simulink model "NUgus"  (R2018a)
settings: Solver=VariableStepAuto  StartTime=0.0  StopTime=inf  RelTol=1e-2
values from neighbouring files (symbols this model uses):
  CM740_acc_bias = 4 * 9.80743    (= 39.22972)    [CM740_init.m]
  CM740_acc_gain = 512 / CM740_acc_centre    [CM740_init.m]
  CM740_gyro_bias = 1600 / 360 * 2 * pi    (= 27.9252680319)    [CM740_init.m]
  CM740_gyro_gain = 512 / CM740_gyro_centre    [CM740_init.m]
  g = 9.8107    [init.m]
  head = [-0.05482228998067195, -0.00010888238321339966, 0.0011712900228573724, 0.41900000000000004]    [comtest.m]
  Kw = 0.9    [init.m]
  model = NUgusKinematics()    [KinematicsTest.m]    (also in Support_Region.m; init.m = NUgusKinematics)
  period = 1.0    (= 1)    [init.m]
  s = mean(abs(present_speed.data))    [RunServoTest.m]
  sample_time = 1/90    (= 0.0111111111111)    [init.m]
  step_height = 0.1    [init.m]
  torso = [0.0050079703254699804, 0.008880921777563762, 0.1021503146237477, 2.5390000000000006]    [comtest.m]
  z0 = 0.45    [init.m]
undefined symbols (not defined in the file or in its folder): sigbuilder_block, X, Y, Z
libraries: sm_lib x206, nesl_utility x82, Contact_Forces_Lib x10
(part 7 of 7)

== system NUgus/NUgus/6 DoF/to IMU ==
  alpha : Inport
  omega : Inport  Port=2
  Rtw : Inport  Port=3
  Data Store Write : DataStoreWrite  DataStoreName=CM740  SampleTime=sample_time  DataStoreElements=CM740.acc_x#CM740.acc_y#CM740.acc_z#CM740.gyro_x#CM740.gyro_y#CM740.gyro_z
  IMU : Subsystem
  wires:
  IMU/3(alphaz) -> Data Store Write/3
  IMU/2(alphay) -> Data Store Write/2
  IMU/1(alphax) -> Data Store Write/1
  IMU/4(omegax) -> Data Store Write/4
  IMU/6(omegaz) -> Data Store Write/6
  Rtw/1 -> IMU/1(Rtw)
  omega/1 -> IMU/2(w)
  alpha/1 -> IMU/3(a)
  IMU/5(omegay) -> Data Store Write/5

== system NUgus/NUgus/IMU1/Convert Acc ==
  PS-Simulink Converter{,1..3} (4 alike) : nesl_utility/PS-Simulink Converter  PhysicalDomain=network_engine_domain  SubClassName=ps_output  LeftPortType=input  RightPortType=output  PseudoPeriodic=off  Frequencies=[]  Unit=1  AffineConversion=off
  Ha : PMIOPort  Side=Left
  x : PMIOPort  Port=2  Side=Left
  y : PMIOPort  Port=3  Side=Left
  z : PMIOPort  Port=4  Side=Left
  Htw : Outport
  ax : Outport  Port=2
  ay : Outport  Port=3
  az : Outport  Port=4
  wires:
  PS-Simulink Converter2/1 -> az/1
  PS-Simulink Converter1/1 -> ay/1
  PS-Simulink Converter/1 -> ax/1
  PS-Simulink Converter3/1 -> Htw/1
  connections:
  PS-Simulink Converter2/LConn1 -- z/RConn1
  PS-Simulink Converter/LConn1 -- x/RConn1
  PS-Simulink Converter1/LConn1 -- y/RConn1
  Ha/RConn1 -- PS-Simulink Converter3/LConn1

== system NUgus/NUgus/IMU1/Convert Gyro ==
  PS-Simulink Converter : nesl_utility/PS-Simulink Converter  PhysicalDomain=network_engine_domain  SubClassName=ps_output  LeftPortType=input  RightPortType=output  PseudoPeriodic=off  Frequencies=[]  Unit=rad/s  AffineConversion=off
  PS-Simulink Converter1 : nesl_utility/PS-Simulink Converter  PhysicalDomain=network_engine_domain  SubClassName=ps_output  LeftPortType=input  RightPortType=output  PseudoPeriodic=off  Frequencies=[]  Unit=rad/s  AffineConversion=off
  PS-Simulink Converter2 : nesl_utility/PS-Simulink Converter  PhysicalDomain=network_engine_domain  SubClassName=ps_output  LeftPortType=input  RightPortType=output  PseudoPeriodic=off  Frequencies=[]  Unit=rad/s  AffineConversion=off
  x : PMIOPort  Side=Left
  y : PMIOPort  Port=2  Side=Left
  z : PMIOPort  Port=3  Side=Left
  wx : Outport
  wy : Outport  Port=2
  wz : Outport  Port=3
  wires:
  PS-Simulink Converter2/1 -> wz/1
  PS-Simulink Converter1/1 -> wy/1
  PS-Simulink Converter/1 -> wx/1
  connections:
  PS-Simulink Converter2/LConn1 -- z/RConn1
  PS-Simulink Converter/LConn1 -- x/RConn1
  PS-Simulink Converter1/LConn1 -- y/RConn1

== system NUgus/NUgus/IMU1/Saturate Acc ==
  Hta : Inport
  Acc : Inport  Port=2
  Acc Saturation : Saturate  UpperLimit=1023  LowerLimit=0
  Add : Sum  Inputs=+++
  Constant : Constant  Value=CM740_acc_bias
  Constant1 : Constant  Value=[0 0 9.80743]
  Gain : Gain  Gain=[0 0 1]
  Gain1 : Gain  Gain=CM740_acc_gain  OutDataTypeStr=int16
  Matrix Multiply : Product  Multiplication=Matrix(*)
  Transpose : Math  Operator=transpose  SaturateOnIntegerOverflow=on
  alpha : Outport
  wires:
  Acc/1 -> Add/3
  Add/1 -> Gain1/1
  Acc Saturation/1 -> alpha/1
  Gain/1 -> Add/1
  Gain1/1 -> Acc Saturation/1
  Constant/1 -> Add/2
  Transpose/1 -> Matrix Multiply/1
  Hta/1 -> Transpose/1
  Constant1/1 -> Matrix Multiply/2
  Matrix Multiply/1 -> Gain/1

== system NUgus/NUgus/IMU1/Saturate Gyro ==
  w : Inport
  Add1 : Sum
  Constant1 : Constant  Value=CM740_gyro_bias
  Gain : Gain  Gain=CM740_gyro_gain  OutDataTypeStr=int16
  Gyro Saturation : Saturate  UpperLimit=1023  LowerLimit=0
  omega : Outport
  wires:
  Constant1/1 -> Add1/2
  Gyro Saturation/1 -> omega/1
  Add1/1 -> Gain/1
  Gain/1 -> Gyro Saturation/1
  w/1 -> Add1/1

== system NUgus/NUgus/left_foot/foot ==
  Inertia : sm_lib/Body Elements/Inertia  InertiaType=Custom  Mass=model.mass.foot(4)  MassUnits=kg  CenterOfMass=[0, 0, 0]  CenterOfMassUnits=m  MomentsOfInertia=[model.inertia.foot(1,1), model.inertia.foot(2,2), model.inertia.foot(3,3)]  MomentsOfInertiaUnits=kg*m^2  ProductsOfInertia=-[model.inertia.foot(2,3), -model.inertia.foot(3,1), -model.inertia.foot(1,2)]  ProductsOfInertiaUnits=kg*m^2  GraphicType=Marker  MarkerShape=Inertia  MarkerSize=20  GraphicVisPropType=SimpleVisualProperties  GraphicDiffuseColor=[0.8 0.8 0.8]  GraphicSpecularColor=[0.5 0.5 0.5 1.0]  GraphicAmbientColor=[0.15 0.15 0.15 1.0]  GraphicEmissiveColor=[0.0 0.0 0.0 1.0]  GraphicShininess=75  GraphicOpacity=inertia_opacity
  InertiaOriginTransform : sm_lib/Frames and Transforms/Rigid Transform  TranslationMethod=Cartesian  TranslationStandardOffset=0  TranslationLengthUnit=m  TranslationStandardAxis=+Z  TranslationCartesianOffset=[-0.007551 -0.077046 -0.031619]  TranslationROffset=0  TranslationROffsetUnits=m  TranslationZOffset=0  TranslationZOffsetUnits=m  TranslationThetaOffset=0  TranslationThetaOffsetUnits=deg  RotationMethod=RotationSequence  RotationAngleUnits=deg  RotationStandardAxis=+Z  RotationAngle=0.0  RotationArbitraryAxis=[0 0 1]  FollAlignAxisA=+X  BaseAlignAxisA=+Y  FollAlignAxisB=+Y  BaseAlignAxisB=+Z  RotationSequenceAxes=BaseAxes  RotationSequence=XYZ  RotationSequenceAngles=[0, 0, 0]  RotationSequenceAnglesUnits=rad  RotationMatrix=[1 0 0; 0 1 0; 0 0 1]
  ReferenceFrame : sm_lib/Frames and Transforms/Reference Frame
  right_ankle_roll_AxisInvTransform : sm_lib/Frames and Transforms/Rigid Transform  TranslationMethod=Cartesian  TranslationStandardOffset=0  TranslationLengthUnit=m  TranslationStandardAxis=+Z  TranslationCartesianOffset=[0, 0, 0]  TranslationROffset=0  TranslationROffsetUnits=m  TranslationZOffset=0  TranslationZOffsetUnits=m  TranslationThetaOffset=0  TranslationThetaOffsetUnits=deg  RotationMethod=ArbitraryAxis  RotationAngleUnits=rad  RotationStandardAxis=+Z  RotationAngle=1.570796326794897  RotationArbitraryAxis=[1, 0, 0]  FollAlignAxisA=+X  BaseAlignAxisA=+Y  FollAlignAxisB=+Y  BaseAlignAxisB=+Z  RotationSequenceAxes=FollowerAxes  RotationSequence=XYX  RotationSequenceAngles=[0 0 0]  RotationSequenceAnglesUnits=deg  RotationMatrix=[1 0 0; 0 1 0; 0 0 1]
  right_foot_visual : sm_lib/Body Elements/Solid  InertiaType=Custom  Mass=0  MassUnits=kg  CenterOfMass=[0, 0, 0]  CenterOfMassUnits=m  MomentsOfInertia=[0, 0, 0]  MomentsOfInertiaUnits=kg*m^2  ProductsOfInertia=[0, 0, 0]  ProductsOfInertiaUnits=kg*m^2  DensityBased=on  Density=1000  DensityUnits=kg/m^3  DoExposeReferenceFrame=on  SerializedFrames=<Frames/>  GraphicType=FromGeometry  MarkerShape=Sphere  MarkerSize=10  GraphicVisPropType=SimpleVisualProperties  GraphicDiffuseColor=[0.5, 0.5, 0.5]  GraphicSpecularColor=[0.5 0.5 0.5 1.0]  GraphicAmbientColor=[0.15 0.15 0.15 1.0]  GraphicEmissiveColor=[0.0 0.0 0.0 1.0]  GraphicShininess=75  GraphicOpacity=1  GeometryShape=FromFile  RectangleSize=[1 1]  RectangleSizeUnits=m  BrickDimensions=[1 1 1]  BrickDimensionUnits=m  CylinderRadius=1  CylinderRadiusUnits=m  CylinderLength=1  CylinderLengthUnits=m  SphereRadius=1  SphereRadiusUnits=m  EllipsoidRadii=[1 1 1]  EllipsoidRadiiUnits=m  ExtrusionCrossSection=[1 1; -1 1; -1 -1; 1 -1]  ExtrusionCrossSectionUnits=m  ExtrusionLength=1  ExtrusionLengthUnits=m  PolygonNumSides=3  PolygonOuterRadius=1  PolygonOuterRadiusUnits=m  ExtGeomFileType=STL  ExtGeomFileName=mesh/left_foot.stl  ExtGeomFileUnits=m  RevolutionCrossSection=[1 1; 1 -1; 2 -1; 2 1]  RevolutionCrossSectionUnits=m  RevolutionExtent=Full  RevolutionAngle=180  RevolutionAngleUnits=deg
  right_foot_visualOriginTransform : sm_lib/Frames and Transforms/Rigid Transform  TranslationMethod=Cartesian  TranslationStandardOffset=0  TranslationLengthUnit=m  TranslationStandardAxis=+Z  TranslationCartesianOffset=[0, 0, 0]  TranslationROffset=0  TranslationROffsetUnits=m  TranslationZOffset=0  TranslationZOffsetUnits=m  TranslationThetaOffset=0  TranslationThetaOffsetUnits=deg  RotationMethod=RotationSequence  RotationAngleUnits=deg  RotationStandardAxis=+Z  RotationAngle=0.0  RotationArbitraryAxis=[0 0 1]  FollAlignAxisA=+X  BaseAlignAxisA=+Y  FollAlignAxisB=+Y  BaseAlignAxisB=+Z  RotationSequenceAxes=BaseAxes  RotationSequence=XYZ  RotationSequenceAngles=[0, 0, 0]  RotationSequenceAnglesUnits=rad  RotationMatrix=[1 0 0; 0 1 0; 0 0 1]
  F : PMIOPort  Side=Left
  B : PMIOPort  Port=2  Side=Right
  connections:
  Inertia/RConn1 -- InertiaOriginTransform/RConn1
  ReferenceFrame/RConn1 -- InertiaOriginTransform/LConn1 -- right_ankle_roll_AxisInvTransform/LConn1 -- right_foot_visualOriginTransform/LConn1 -- B/RConn1
  right_ankle_roll_AxisInvTransform/RConn1 -- F/RConn1
  right_foot_visual/RConn1 -- right_foot_visualOriginTransform/RConn1

== system NUgus/NUgus/right_foot/foot ==
  Inertia : sm_lib/Body Elements/Inertia  InertiaType=Custom  Mass=model.mass.foot(4)  MassUnits=kg  CenterOfMass=[0, 0, 0]  CenterOfMassUnits=m  MomentsOfInertia=[model.inertia.foot(1,1), model.inertia.foot(2,2), model.inertia.foot(3,3)]  MomentsOfInertiaUnits=kg*m^2  ProductsOfInertia=-[model.inertia.foot(2,3), model.inertia.foot(3,1), model.inertia.foot(1,2)]  ProductsOfInertiaUnits=kg*m^2  GraphicType=Marker  MarkerShape=Inertia  MarkerSize=20  GraphicVisPropType=SimpleVisualProperties  GraphicDiffuseColor=[0.8 0.8 0.8]  GraphicSpecularColor=[0.5 0.5 0.5 1.0]  GraphicAmbientColor=[0.15 0.15 0.15 1.0]  GraphicEmissiveColor=[0.0 0.0 0.0 1.0]  GraphicShininess=75  GraphicOpacity=inertia_opacity
  InertiaOriginTransform : sm_lib/Frames and Transforms/Rigid Transform  TranslationMethod=Cartesian  TranslationStandardOffset=0  TranslationLengthUnit=m  TranslationStandardAxis=+Z  TranslationCartesianOffset=[-0.007551 -0.077046 -0.031619]  TranslationROffset=0  TranslationROffsetUnits=m  TranslationZOffset=0  TranslationZOffsetUnits=m  TranslationThetaOffset=0  TranslationThetaOffsetUnits=deg  RotationMethod=RotationSequence  RotationAngleUnits=deg  RotationStandardAxis=+Z  RotationAngle=0.0  RotationArbitraryAxis=[0 0 1]  FollAlignAxisA=+X  BaseAlignAxisA=+Y  FollAlignAxisB=+Y  BaseAlignAxisB=+Z  RotationSequenceAxes=BaseAxes  RotationSequence=XYZ  RotationSequenceAngles=[0, 0, 0]  RotationSequenceAnglesUnits=rad  RotationMatrix=[1 0 0; 0 1 0; 0 0 1]
  ReferenceFrame : sm_lib/Frames and Transforms/Reference Frame
  right_ankle_roll_AxisInvTransform : sm_lib/Frames and Transforms/Rigid Transform  TranslationMethod=Cartesian  TranslationStandardOffset=0  TranslationLengthUnit=m  TranslationStandardAxis=+Z  TranslationCartesianOffset=[0, 0, 0]  TranslationROffset=0  TranslationROffsetUnits=m  TranslationZOffset=0  TranslationZOffsetUnits=m  TranslationThetaOffset=0  TranslationThetaOffsetUnits=deg  RotationMethod=ArbitraryAxis  RotationAngleUnits=rad  RotationStandardAxis=+Z  RotationAngle=1.570796326794897  RotationArbitraryAxis=[1, 0, 0]  FollAlignAxisA=+X  BaseAlignAxisA=+Y  FollAlignAxisB=+Y  BaseAlignAxisB=+Z  RotationSequenceAxes=FollowerAxes  RotationSequence=XYX  RotationSequenceAngles=[0 0 0]  RotationSequenceAnglesUnits=deg  RotationMatrix=[1 0 0; 0 1 0; 0 0 1]
  right_foot_visual : sm_lib/Body Elements/Solid  InertiaType=Custom  Mass=0  MassUnits=kg  CenterOfMass=[0, 0, 0]  CenterOfMassUnits=m  MomentsOfInertia=[0, 0, 0]  MomentsOfInertiaUnits=kg*m^2  ProductsOfInertia=[0, 0, 0]  ProductsOfInertiaUnits=kg*m^2  DensityBased=on  Density=1000  DensityUnits=kg/m^3  DoExposeReferenceFrame=on  SerializedFrames=<Frames/>  GraphicType=FromGeometry  MarkerShape=Sphere  MarkerSize=10  GraphicVisPropType=SimpleVisualProperties  GraphicDiffuseColor=[0.5, 0.5, 0.5]  GraphicSpecularColor=[0.5 0.5 0.5 1.0]  GraphicAmbientColor=[0.15 0.15 0.15 1.0]  GraphicEmissiveColor=[0.0 0.0 0.0 1.0]  GraphicShininess=75  GraphicOpacity=1  GeometryShape=FromFile  RectangleSize=[1 1]  RectangleSizeUnits=m  BrickDimensions=[1 1 1]  BrickDimensionUnits=m  CylinderRadius=1  CylinderRadiusUnits=m  CylinderLength=1  CylinderLengthUnits=m  SphereRadius=1  SphereRadiusUnits=m  EllipsoidRadii=[1 1 1]  EllipsoidRadiiUnits=m  ExtrusionCrossSection=[1 1; -1 1; -1 -1; 1 -1]  ExtrusionCrossSectionUnits=m  ExtrusionLength=1  ExtrusionLengthUnits=m  PolygonNumSides=3  PolygonOuterRadius=1  PolygonOuterRadiusUnits=m  ExtGeomFileType=STL  ExtGeomFileName=mesh/right_foot.stl  ExtGeomFileUnits=m  RevolutionCrossSection=[1 1; 1 -1; 2 -1; 2 1]  RevolutionCrossSectionUnits=m  RevolutionExtent=Full  RevolutionAngle=180  RevolutionAngleUnits=deg
  right_foot_visualOriginTransform : sm_lib/Frames and Transforms/Rigid Transform  TranslationMethod=Cartesian  TranslationStandardOffset=0  TranslationLengthUnit=m  TranslationStandardAxis=+Z  TranslationCartesianOffset=[0, 0, 0]  TranslationROffset=0  TranslationROffsetUnits=m  TranslationZOffset=0  TranslationZOffsetUnits=m  TranslationThetaOffset=0  TranslationThetaOffsetUnits=deg  RotationMethod=RotationSequence  RotationAngleUnits=deg  RotationStandardAxis=+Z  RotationAngle=0.0  RotationArbitraryAxis=[0 0 1]  FollAlignAxisA=+X  BaseAlignAxisA=+Y  FollAlignAxisB=+Y  BaseAlignAxisB=+Z  RotationSequenceAxes=BaseAxes  RotationSequence=XYZ  RotationSequenceAngles=[0, 0, 0]  RotationSequenceAnglesUnits=rad  RotationMatrix=[1 0 0; 0 1 0; 0 0 1]
  F : PMIOPort  Side=Left
  B : PMIOPort  Port=2  Side=Right
  connections:
  Inertia/RConn1 -- InertiaOriginTransform/RConn1
  ReferenceFrame/RConn1 -- InertiaOriginTransform/LConn1 -- B/RConn1 -- right_ankle_roll_AxisInvTransform/LConn1 -- right_foot_visualOriginTransform/LConn1
  right_ankle_roll_AxisInvTransform/RConn1 -- F/RConn1
  right_foot_visual/RConn1 -- right_foot_visualOriginTransform/RConn1

== system NUgus/NUgus/6 DoF/to IMU/IMU ==
  Rtw : Inport
  w : Inport  Port=2
  a : Inport  Port=3
  Demux : Demux  Outputs=3
  Demux1 : Demux  Outputs=3
  IMU Continuous : Scope  NumInputPorts=2
  IMU Discrete : Scope  NumInputPorts=2
  Saturate Acc : Subsystem
  Saturate Gyro : Subsystem
  alphax : Outport
  alphay : Outport  Port=2
  alphaz : Outport  Port=3
  omegax : Outport  Port=4
  omegay : Outport  Port=5
  omegaz : Outport  Port=6
  wires:
  Demux/1 -> omegax/1
  Demux/2 -> omegay/1
  Demux/3 -> omegaz/1
  Demux1/3 -> alphaz/1
  Demux1/1 -> alphax/1
  Demux1/2 -> alphay/1
  Saturate Acc/1(alpha) -> IMU Discrete/2, Demux1/1
  w/1 -> IMU Continuous/1, Saturate Gyro/1(w)
  Saturate Gyro/1(omega) -> IMU Discrete/1, Demux/1
  a/1 -> Saturate Acc/2(Acc), IMU Continuous/2
  Rtw/1 -> Saturate Acc/1(Rtw)

== system NUgus/NUgus/6 DoF/to IMU/IMU/Saturate Acc ==
  Rtw : Inport
  Acc : Inport  Port=2
  Acc Saturation : Saturate  UpperLimit=1023  LowerLimit=0
  Add : Sum  Inputs=+++
  Constant : Constant  Value=CM740_acc_bias
  Constant1 : Constant  Value=[0 0 9.80743]
  Gain : Gain  Gain=[1 1 -1]
  Gain1 : Gain  Gain=CM740_acc_gain  OutDataTypeStr=int16
  Matrix Multiply : Product  Multiplication=Matrix(*)
  Transpose : Math  Operator=transpose  SaturateOnIntegerOverflow=on
  alpha : Outport
  wires:
  Acc/1 -> Add/3
  Add/1 -> Gain1/1
  Acc Saturation/1 -> alpha/1
  Gain/1 -> Add/1
  Gain1/1 -> Acc Saturation/1
  Constant/1 -> Add/2
  Transpose/1 -> Matrix Multiply/1
  Rtw/1 -> Transpose/1
  Constant1/1 -> Matrix Multiply/2
  Matrix Multiply/1 -> Gain/1

== system NUgus/NUgus/6 DoF/to IMU/IMU/Saturate Gyro ==
  w : Inport
  Add1 : Sum
  Constant1 : Constant  Value=CM740_gyro_bias
  Gain : Gain  Gain=CM740_gyro_gain  OutDataTypeStr=int16
  Gyro Saturation : Saturate  UpperLimit=1023  LowerLimit=0
  omega : Outport
  wires:
  Constant1/1 -> Add1/2
  Gyro Saturation/1 -> omega/1
  Add1/1 -> Gain/1
  Gain/1 -> Gyro Saturation/1
  w/1 -> Add1/1

== matlab function NUgus/Kinematics/Forward Kinematics/Simulink Function/FK Function ==
  data: HtRSp output; p input; HtLSp output; HtRSr output; HtLSr output; HtRE output; HtLE output; HtRHy output; HtLHy output; HtRHr output; HtLHr output; HtRHp output; HtLHp output; HtRK output; HtLK output; HtRAp output; HtLAp output; HtRAr output; HtLAr output; HtHy output; HtHp output
function [HtRSp, HtLSp, HtRSr, HtLSr, HtRE, HtLE, HtRHy, HtLHy, HtRHr, HtLHr, HtRHp, HtLHp, HtRK, HtLK, HtRAp, HtLAp, HtRAr, HtLAr, HtHy, HtHp] = FK(p)
    model = NUgusKinematics();

    kinematics = Kinematics(model);
    
    % Get FK for arms
    [RSp, RSr, RE] = kinematics.armFK(p, false);
    [LSp, LSr, LE] = kinematics.armFK(p, true);
    % Get FK for legs
    [RHy, RHr, RHp, RK, RAp, RAr] = kinematics.legFK(p, false);
    [LHy, LHr, LHp, LK, LAp, LAr] = kinematics.legFK(p, true);
    % Get FK for Head
    [Hy, Hp] = kinematics.headFK(p);
    
    % Return FK in servo order
    HtRSp = RSp.tf;
    HtLSp = LSp.tf;
    
    HtRSr = RSr.tf;
    HtLSr = LSr.tf;
    
    HtRE = RE.tf;
    HtLE = LE.tf;
    
    HtRHy = RHy.tf;
    HtLHy = LHy.tf;
    
    HtRHr = RHr.tf;
    HtLHr = LHr.tf;
    
    HtRHp = RHp.tf;
    HtLHp = LHp.tf;
    
    HtRK = RK.tf;
    HtLK = LK.tf;
    
    HtRAp = RAp.tf;
    HtLAp = LAp.tf;
    
    HtRAr = RAr.tf;
    HtLAr = LAr.tf;
    
    HtHy = Hy.tf;
    HtHp = Hp.tf;
end

== matlab function NUgus/Kinematics/Centre of Mass/Simulink Function/COM Function ==
  data: HtRSp input; HtLSp input; HtRSr input; HtLSr input; HtRE input; HtLE input; HtRHy input; HtLHy input; HtRHr input; HtLHr input; HtRHp input; HtLHp input; HtRK input; HtLK input; HtRAp input; HtLAp input; HtRAr input; HtLAr input; HtHy input; HtHp input; com output; mass output
function [com, mass] = COM(HtRSp, HtLSp, HtRSr, HtLSr, HtRE, HtLE, HtRHy, HtLHy, HtRHr, HtLHr, HtRHp, HtLHp, HtRK, HtLK, HtRAp, HtLAp, HtRAr, HtLAr, HtHy, HtHp)
    model = NUgusKinematics();
    
    % Store mass particles and their transforms to multiply
    ms = [model.mass.head; model.mass.arm_upper; model.mass.arm_upper; model.mass.arm_lower; model.mass.arm_lower; model.mass.hip_block; model.mass.hip_block; model.mass.leg_upper; model.mass.leg_upper; model.mass.leg_lower; model.mass.leg_lower; model.mass.ankle_block; model.mass.ankle_block; model.mass.foot; model.mass.foot; model.mass.torso];
    tf = [HtHp, HtRSp, HtLSp, HtRSr, HtLSr, HtRHr, HtLHr, HtRHp, HtLHp, HtRK, HtLK, HtRAp, HtLAp, HtRAr, HtLAr, [1 0 0 0; 0 1 0 0; 0 0 1 0; 0 0 0 1]];

    % Store CoM as x,y,z coordinates
    com = [0; 0; 0];
    mass = 0;

    for ii=1:size(ms, 1)
        % Get transform of the particle
        t = tf(1:4, ii*4-3:ii*4);
        % Alias particle CoM and mass for convenience
        p_com  = [ms(ii, 1:3) 1]';
        p_com  = t * p_com;
        p_mass = ms(ii, 4);
        % Calculate new CoM and updated mass
        com = (com * mass + p_com(1:3) * p_mass) / (mass + p_mass);
        mass = mass + p_mass;
    end
    
end

== matlab function NUgus/Simulink Function/MATLAB Function ==
  data: x input; H output; y input; z input; roll input; pitch input; yaw input
function H = getTransform(x,y,z,roll,pitch,yaw)
    t = Transform3D();    
    t = t.translate([x,y,z]).rotateX(roll).rotateY(pitch).rotateZ(yaw);
    H = t.tf;
end

== matlab function NUgus/Kinematics/Inverse Kinematics/Simulink Function/IK Function ==
  data: thetaTRSp output; rTRh input; rTLh input; HTRl input; HTLl input; rCP input; thetaTLSp output; thetaTRSr output; thetaTLSr output; thetaTRE output; thetaTLE output; thetaTRHy output; thetaTLHy output; thetaTRHr output; thetaTLHr output; thetaTRHp output; thetaTLHp output; thetaTRK output; thetaTLK output; thetaTRAp output; thetaTLAp output; thetaTRAr output; thetaTLAr output; thetaTNy output; thetaTNp output
function [thetaTRSp, thetaTLSp, thetaTRSr, thetaTLSr, thetaTRE, thetaTLE, thetaTRHy, thetaTLHy, thetaTRHr, thetaTLHr, thetaTRHp, thetaTLHp, thetaTRK, thetaTLK, thetaTRAp, thetaTLAp, thetaTRAr, thetaTLAr, thetaTNy, thetaTNp] = IK(rTRh, rTLh, HTRl, HTLl, rCP)
    model = NUgusKinematics();

    kinematics = Kinematics(model);

    % Head IK
    [thetaTNy, thetaTNp] = kinematics.headIK(rCP);
    
    % Arm IK
    [thetaTRSp, thetaTRSr, thetaTRE] = kinematics.armIK(rTRh, false);
    [thetaTLSp, thetaTLSr, thetaTLE] = kinematics.armIK(rTLh, true);
    
    % Leg IK
    [thetaTRHy, thetaTRHr, thetaTRHp, thetaTRK, thetaTRAp, thetaTRAr] = kinematics.legIK(HTRl, false);
    [thetaTLHy, thetaTLHr, thetaTLHp, thetaTLK, thetaTLAp, thetaTLAr] = kinematics.legIK(HTLl, true);
end

== stateflow chart NUgus/Control/Step Logic ==
  settings: updateMethod=DISCRETE  sampleTime=0.1  initializeOutput=1
  state update [function]
    (default) -> (junction 109) : {
        | %Update right
        | xr = xr + Kw*(xr_ref - xr);
        | yr = yr + Kw*(yr_ref - yr);
        | zr = zr + Kw*(zr_ref - zr);
        | % Update left
        | xl = xl + Kw*(xl_ref - xl);
        | yl = yl + Kw*(yl_ref - yl);
        | zl = zl + Kw*(zl_ref - zl);
        | % Store updates
        | rfoot = [xr; yr; zr];
        | lfoot = [xl; yl; zl];
        | }
  state RightSwing
    % Right foot swing
    % Left foot support
    en, du:
    update;
    state Right [parallel]
      en,du:
      % Left support
      zl_ref = zLow;
      % Right swing
      xr_ref = xin;
      yr_ref = min(-0.1,yin);
      zr_ref = zHigh;
      on after(0.5*period, sec):
      zr_ref = zLow;
      settings: executionOrder=1
    state Left [parallel]
      en,du:
      % Set x,y coords for support
      xl_ref = -xr_ref;
      yl_ref = max(0.1, yin);
      hrl_ref = -atan2(xl_ref, step_height);
      settings: executionOrder=2
  state LeftSwing
    % Left foot swing
    % Right foot support
    en, du:
    update;
    state Right [parallel]
      en,du:
      % Set x,y coords for support
      xr_ref = -xl_ref;
      yr_ref = min(-0.1, yin);
      hrr_ref = -atan2(2*xl_ref, step_height);
      settings: executionOrder=1
    state Left [parallel]
      en,du:
      % Right support
      zr_ref = zLow;
      % Left swing
      xl_ref = xin;
      yl_ref = max(0.1, yin);
      zl_ref = zHigh;
      on after(0.5*period, sec):
      zl_ref = zLow;
      settings: executionOrder=2
  (default) -> RightSwing : % Initialise
      | {
      | zLow = -z0;
      | zHigh = -z0 + step_height;
      | % Initialise foot positions
      | xr = 0; yr = -0.1; zr = zLow;
      | xl = 0; yl = 0.1; zl = zLow;
      | % Initialise reference positions
      | xr_ref = 0; yr_ref = -0.1; zr_ref = zLow;
      | xl_ref = 0; yl_ref = 0.1; zl_ref = zLow;
      | }
  RightSwing -> LeftSwing : [after(period, sec)]
  LeftSwing -> RightSwing : [after(period, sec)]
  data: com input size=[1, 3]; Htw input size=[4, 4]; rfoot output size=[3]; lfoot output size=[3]; period parameter double; xin input double; xl local; yl local; zl_ref local; yl_ref local; xr local; zr_ref local; yr_ref local; zl local; yr local; zr local; zLow local; zHigh local; xl_ref local; xr_ref local; Kw parameter double; yin input; step_height parameter double; z0 parameter double; hrl_ref output; hrr_ref output

== matlab function NUgus/6 DoF/MATLAB Function ==
  data: m input; h output; p input
function h = hom(m, p)
    h = [m p; [0 0 0 1]];
end

== matlab function NUgus/Kinematics/Torso Centre of Mass/Simulink Function/MATLAB Function ==
  data: HtRSp input; torso_com output; HtLSp input; HtRSr input; HtLSr input; HtRE input; HtLE input; HtHy input; HtHp input; torso_mass output
function [torso_com, torso_mass] = TorsoCOM(HtRSp, HtLSp, HtRSr, HtLSr, HtRE, HtLE, HtHy, HtHp)
    model = NUgusKinematics();
    
    % Store mass particles and their transforms to multiply
    ms = [model.mass.head; model.mass.arm_upper; model.mass.arm_upper; model.mass.arm_lower; model.mass.arm_lower; model.mass.torso];
    tf = [HtHp, HtRSp, HtLSp, HtRSr, HtLSr, [1 0 0 0; 0 1 0 0; 0 0 1 0; 0 0 0 1]];

    % Store CoM as x,y,z coordinates
    torso_com = [0; 0; 0];
    torso_mass = 0;

    for ii=1:size(ms, 1)
        % Get transform of the particle
        t = tf(1:4, ii*4-3:ii*4);
        % Alias particle CoM and mass for convenience
        p_com  = [ms(ii, 1:3) 1]';
        p_com  = t * p_com;
        p_mass = ms(ii, 4);
        % Calculate new CoM and updated mass
        torso_com = (torso_com * torso_mass + p_com(1:3) * p_mass) / (torso_mass + p_mass);
        torso_mass = torso_mass + p_mass;
    end
    
end

== matlab function NUgus/Kinematics/MATLAB Function ==
  data: pitch output; torso_com input; HtRAr input; roll output; HtLAr input; Htw input
function [pitch, roll] = SupportCOM(torso_com, HtRAr, HtLAr, Htw)
    % Get desired position of CoM between supporting feet
    com = Htw * ((HtRAr(:, 4) + HtLAr(:,4)) / 2);
    
    % Get vector between current torso CoM and desired CoM in world space
    v = (Htw * [torso_com 1]') - com;
    
    roll  = atan(v(2) / com(3));
    pitch = atan(v(1) / com(3));
end

== stateflow chart NUgus/Control/Capture ==
  state update [function]
    (default) -> (junction 6) : {
        | %Update right
        | xr = xr + Kw*(xr_ref - xr);
        | yr = yr + Kw*(yr_ref - yr);
        | zr = zr + Kw*(zr_ref - zr);
        | % Update left
        | xl = xl + Kw*(xl_ref - xl);
        | yl = yl + Kw*(yl_ref - yl);
        | zl = zl + Kw*(zl_ref - zl);
        | % Store updates
        | rfoot = [xr; yr; zr];
        | lfoot = [xl; yl; zl];
        | % Calculate distance to ZMP point
        | dzmp = sqrt((zmpx - comx) ^ 2 + (zmpy - comy) ^ 2);
        | }
  state init
    en,du:
    update;
  state RightSwing
    % Right foot swing
    % Left foot support
    en, du:
    update;
    state Right [parallel]
      en,du:
      % Left support
      zl_ref = zLow;
      % Right swing
      xr_ref = zmpx;
      yr_ref = min(-0.1, zmpy);
      zr_ref = zHigh;
      settings: executionOrder=1
    state Left [parallel]
      en,du:
      % Set x,y coords for support
      xl_ref = -xr_ref;
      yl_ref = max(0.1, zmpy);
      settings: executionOrder=2
  state LeftSwing
    % Left foot swing
    % Right foot support
    en, du:
    update;
    state Right [parallel]
      en,du:
      % Set x,y coords for support
      xr_ref = -xl_ref;
      yr_ref = min(-0.1, zmpy);
      settings: executionOrder=2
    state Left [parallel]
      en,du:
      % Right support
      zr_ref = zLow;
      % Left swing
      xl_ref = zmpx;
      yl_ref = max(0.1, zmpy);
      zl_ref = zHigh;
      settings: executionOrder=1
  (default) -> init : % Initialise
      | {
      | zLow = -z0;
      | zHigh = -z0 + step_height;
      | % Initialise foot positions
      | xr = 0; yr = -0.1; zr = zLow;
      | xl = 0; yl = 0.1; zl = zLow;
      | % Initialise reference positions
      | xr_ref = 0; yr_ref = -0.1; zr_ref = zLow;
      | xl_ref = 0; yl_ref = 0.1; zl_ref = zLow;
      | }
  RightSwing -> init : [dzmp < 0.1]{zr_ref = zLow;}
  LeftSwing -> init : [dzmp <= 0.1]{xl_ref = 0; yl_ref = 0.1; zl_ref = zLow;}
  init -> (junction 18) : [dzmp > 0.2]
  (junction 18) -> LeftSwing [order 2]
  (junction 18) -> RightSwing [order 1] : [zmpy < 0]
  data: zmpx input; zmpy input; dzmp local; period parameter; z0 parameter; step_height parameter; zl_ref local; zr_ref local; xl local; zr local; yr_ref local; xr local; yr local; yl_ref local; zl local; yl local; zHigh local; xr_ref local; xl_ref local; zLow local; rfoot output; lfoot output; Kw parameter; comx input; comy input

== matlab function NUgus/Control/Ground Space ==
  data: Htf input; Htg output; Htw input
function Htg = GroundSpace(Htf, Htw)
    Rwf = Htw(1:3,1:3) * Htf(1:3, 1:3);
    % Get angle to rotate about axis
    alpha = acos(max(min(Rwf(3,3), 1), -1));
    % Get normalised axis
    axis = cross(Rwf(1:3, 3), [0 0 1]);
    axis = axis / (sqrt(axis(1) ^ 2 + axis(2) ^ 2 + axis(3) ^ 2));

    % Alias for convenience
    calpha = cos(alpha);
    salpha = sin(alpha);
    % Create angle, axis rotation matrix
    Rwg = [calpha+(1-calpha)*axis(1)^2              (1-calpha)*axis(1)*axis(2)-axis(3)*salpha  (1-calpha)*axis(1)*axis(3) + axis(2)*salpha;...
         (1-calpha)*axis(2)*axis(1)+axis(3)*salpha  calpha + (1-calpha)*axis(2)^2              (1-calpha)*axis(2)*axis(3)-axis(1)*salpha;...
         (1-calpha)*axis(3)*axis(1)-axis(2)*salpha  (1-calpha)*axis(3)*axis(2)+axis(1)*salpha  calpha+(1-calpha)*axis(3)^2];
    
    % Create homogeneous transform from ground to torso
    Htg = eye(4);
    % Rotation
    Htg(1:3,1:3) = Htw(1:3,1:3)' * Rwg;
    % Translation
    Htg(1:3,4) = Htf(1:3, 4);
end
